simulink model "Simple_Pendulum"  (R2023b)
settings: Solver=VariableStepAuto  StartTime=0.0  StopTime=10.0  RelTol=1e-3
values from neighbouring files (symbols this model uses):
  g = 9.81    [Simple_Pendulum_parameters.m]
undefined symbols (not defined in the file or in its folder): angular_theta, L
settings Model: Creator=DELL  LastModifiedBy=DELL

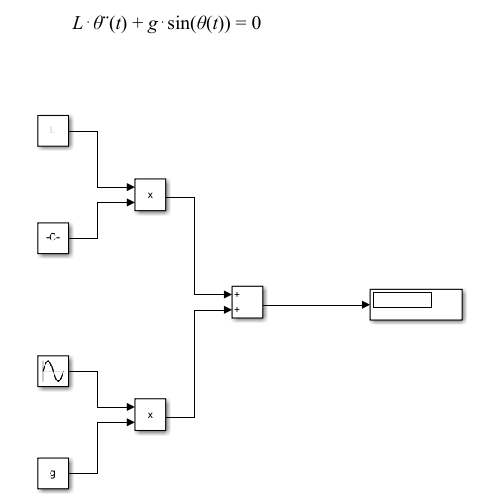
[thumbnail: Simulink's stored preview of the top-level diagram]
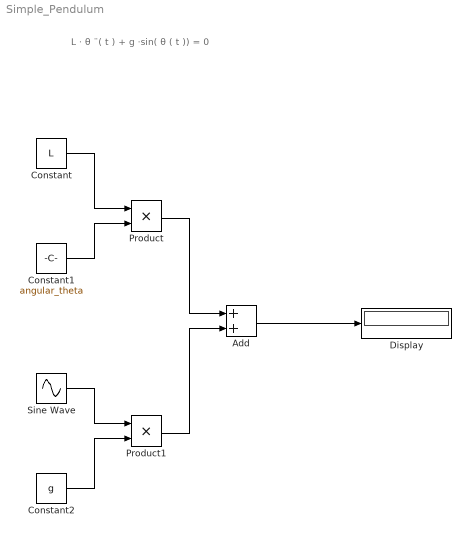
== system Simple_Pendulum ==
  note: L ⋅ θ ¨( t ) + g ⋅sin( θ ( t )) = 0
  Add : Sum
  Constant : Constant  Value=L
  Constant1 : Constant  Value=angular_theta
  Constant2 : Constant  Value=g
  Display : Display
  Product : Product
  Product1 : Product
  Sine Wave : Sin  SampleTime=0
  wires:
  Constant/1 -> Product/1
  Constant1/1 -> Product/2
  Sine Wave/1 -> Product1/1
  Constant2/1 -> Product1/2
  Product/1 -> Add/1
  Product1/1 -> Add/2
  Add/1 -> Display/1
